simulink library "plant_bench_lib"  (R2022b)
settings: Solver=VariableStepAuto  StartTime=0.0  StopTime=10.0  RelTol=1e-3
libraries: AMK_CAN_lib x1
settings Model: Creator=dr_pa  LastModifiedBy=dr_pa

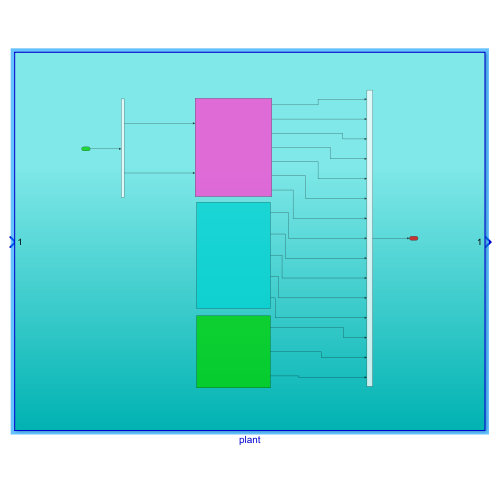
[thumbnail: Simulink's stored preview of the top-level diagram]
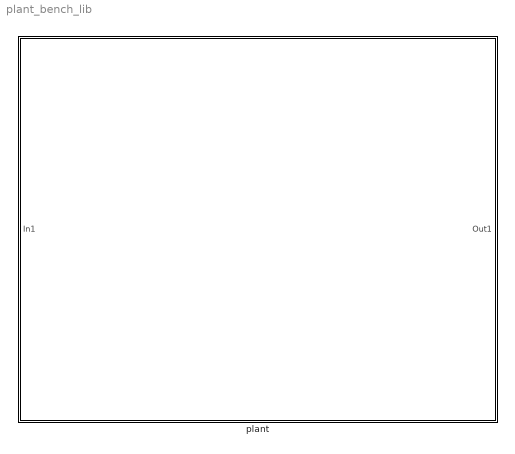
== system plant_bench_lib ==
  plant : Subsystem

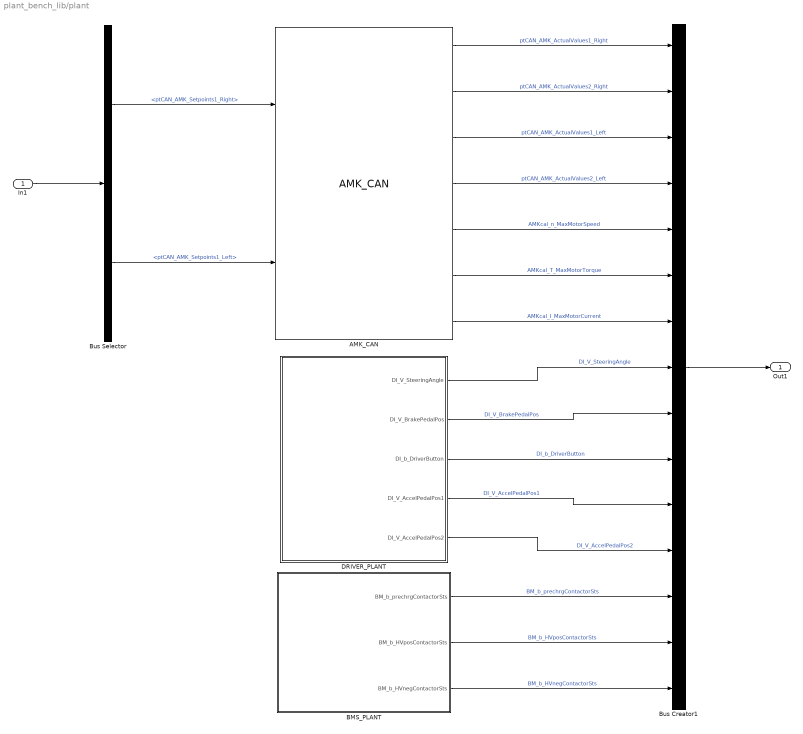
== system plant_bench_lib/plant ==
  In1 : Inport
  AMK_CAN : AMK_CAN_lib/AMK_CAN  SystemSampleTime=-1  VariantActivationTime=update diagram  Latency=0  AutoFrameSizeCalculation=off
  BMS_PLANT : Subsystem
  Bus Creator1 : BusCreator  Inputs=15
  Bus Selector : BusSelector  OutputSignals=ptCAN_AMK_Setpoints1_Right,ptCAN_AMK_Setpoints1_Left
  DRIVER_PLANT : Subsystem
  Out1 : Outport
  wires:
  DRIVER_PLANT/2(DI_V_BrakePedalPos) -> Bus Creator1/9  "DI_V_BrakePedalPos"
  AMK_CAN/2 -> Bus Creator1/2  "ptCAN_AMK_ActualValues2_Right"
  BMS_PLANT/3(BM_b_HVnegContactorSts) -> Bus Creator1/15  "BM_b_HVnegContactorSts"
  AMK_CAN/4 -> Bus Creator1/4  "ptCAN_AMK_ActualValues2_Left"
  Bus Creator1/1 -> Out1/1
  AMK_CAN/1 -> Bus Creator1/1  "ptCAN_AMK_ActualValues1_Right"
  DRIVER_PLANT/1(DI_V_SteeringAngle) -> Bus Creator1/8  "DI_V_SteeringAngle"
  BMS_PLANT/2(BM_b_HVposContactorSts) -> Bus Creator1/14  "BM_b_HVposContactorSts"
  DRIVER_PLANT/3(DI_b_DriverButton) -> Bus Creator1/10  "DI_b_DriverButton"
  DRIVER_PLANT/5(DI_V_AccelPedalPos2) -> Bus Creator1/12  "DI_V_AccelPedalPos2"
  DRIVER_PLANT/4(DI_V_AccelPedalPos1) -> Bus Creator1/11  "DI_V_AccelPedalPos1"
  BMS_PLANT/1(BM_b_prechrgContactorSts) -> Bus Creator1/13  "BM_b_prechrgContactorSts"
  AMK_CAN/3 -> Bus Creator1/3  "ptCAN_AMK_ActualValues1_Left"
  In1/1 -> Bus Selector/1
  Bus Selector/1 -> AMK_CAN/1  "<ptCAN_AMK_Setpoints1_Right>"
  Bus Selector/2 -> AMK_CAN/2  "<ptCAN_AMK_Setpoints1_Left>"
  AMK_CAN/5 -> Bus Creator1/5  "AMKcal_n_MaxMotorSpeed"
  AMK_CAN/6 -> Bus Creator1/6  "AMKcal_T_MaxMotorTorque"
  AMK_CAN/7 -> Bus Creator1/7  "AMKcal_I_MaxMotorCurrent"

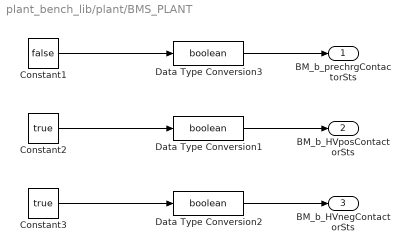
== system plant_bench_lib/plant/BMS_PLANT ==
  Constant1 : Constant  Value=false  OutDataTypeStr=boolean
  Constant2 : Constant  Value=true  OutDataTypeStr=boolean
  Constant3 : Constant  Value=true  OutDataTypeStr=boolean
  Data Type Conversion1 : DataTypeConversion  OutDataTypeStr=boolean  SaturateOnIntegerOverflow=off  RndMeth=Floor
  Data Type Conversion2 : DataTypeConversion  OutDataTypeStr=boolean  SaturateOnIntegerOverflow=off  RndMeth=Floor
  Data Type Conversion3 : DataTypeConversion  OutDataTypeStr=boolean  SaturateOnIntegerOverflow=off  RndMeth=Floor
  BM_b_prechrgContactorSts : Outport
  BM_b_HVposContactorSts : Outport  Port=2
  BM_b_HVnegContactorSts : Outport  Port=3
  wires:
  Constant1/1 -> Data Type Conversion3/1
  Data Type Conversion3/1 -> BM_b_prechrgContactorSts/1
  Constant2/1 -> Data Type Conversion1/1
  Data Type Conversion1/1 -> BM_b_HVposContactorSts/1
  Data Type Conversion2/1 -> BM_b_HVnegContactorSts/1
  Constant3/1 -> Data Type Conversion2/1

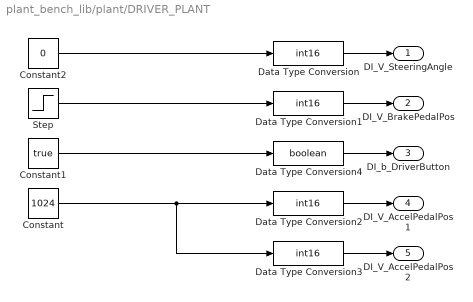
== system plant_bench_lib/plant/DRIVER_PLANT ==
  Constant : Constant  Value=1024
  Constant1 : Constant  Value=true  OutDataTypeStr=boolean
  Constant2 : Constant  Value=0
  Data Type Conversion{,1..3} (4 alike) : DataTypeConversion  OutDataTypeStr=int16  SaturateOnIntegerOverflow=off  RndMeth=Floor
  Data Type Conversion4 : DataTypeConversion  OutDataTypeStr=boolean  SaturateOnIntegerOverflow=off  RndMeth=Floor
  Step : Step  Time=2  Before=75  After=0  OutDataTypeStr=single  SampleTime=0
  DI_V_SteeringAngle : Outport
  DI_V_BrakePedalPos : Outport  Port=2
  DI_b_DriverButton : Outport  Port=3
  DI_V_AccelPedalPos1 : Outport  Port=4
  DI_V_AccelPedalPos2 : Outport  Port=5
  wires:
  Step/1 -> Data Type Conversion1/1
  Constant1/1 -> Data Type Conversion4/1
  Constant/1 -> Data Type Conversion3/1, Data Type Conversion2/1
  Constant2/1 -> Data Type Conversion/1
  Data Type Conversion/1 -> DI_V_SteeringAngle/1
  Data Type Conversion4/1 -> DI_b_DriverButton/1
  Data Type Conversion1/1 -> DI_V_BrakePedalPos/1
  Data Type Conversion2/1 -> DI_V_AccelPedalPos1/1
  Data Type Conversion3/1 -> DI_V_AccelPedalPos2/1
